simulink model "blocco"  (R2020b)
settings: Solver=VariableStepAuto  StartTime=0.0  StopTime=10.0  RelTol=1e-3
values from neighbouring files (symbols this model uses):
  Beq_hat = 1.07084792335e-06    [params_estimated_LAB0.mat]
  daq =     [params_inertial_case.mat]    (also in params_resonant_case.mat)
  drv =     [params_inertial_case.mat]    (also in params_resonant_case.mat)
  gbox =     [params_inertial_case.mat]    (also in params_resonant_case.mat)
  Jeq_hat = 8.03522579674e-07    [params_estimated_LAB0.mat]
  mot =     [params_inertial_case.mat]    (also in params_resonant_case.mat)
  rads2rpm = 9.54929658551    [params_inertial_case.mat]    (also in params_resonant_case.mat)
  sens =     [params_inertial_case.mat]    (also in params_resonant_case.mat)
  tau_hat = 0.00714370660323    [params_estimated_LAB0.mat]
undefined symbols (not defined in the file or in its folder): ctrl, deg2V, den, pulse2deg, s, V2deg
settings Model: Creator=39345  LastModifiedBy=39345

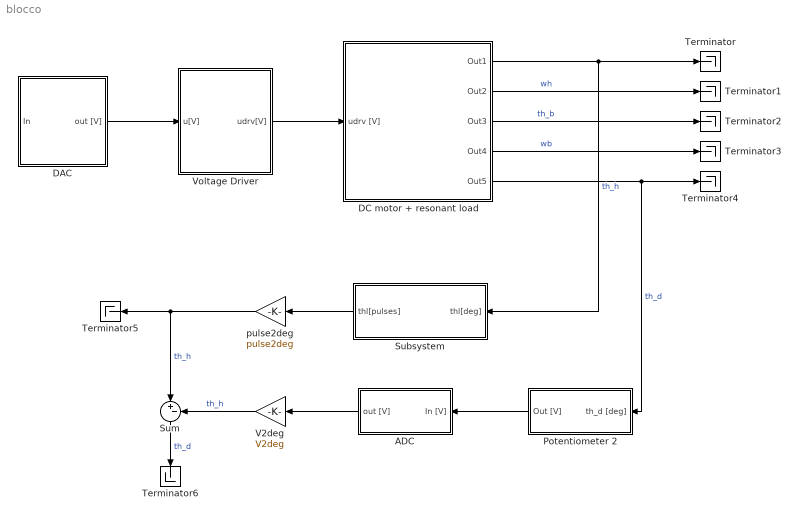
== system blocco ==
  ADC : Subsystem
  DAC : Subsystem
  DC motor + resonant load : Subsystem
  Potentiometer 2 : Subsystem
  Subsystem : Subsystem
  Sum : Sum  Inputs=|+-
  Terminator{,1..6} (7 alike) : Terminator
  V2deg : Gain  Gain=V2deg
  Voltage Driver : Subsystem
  pulse2deg : Gain  Gain=pulse2deg
  wires:
  DC motor + resonant load/1(Out1) -> Subsystem/1(thl[deg]), Terminator/1  "th_h"
  DC motor + resonant load/2(Out2) -> Terminator1/1  "wh"
  DC motor + resonant load/3(Out3) -> Terminator2/1  "th_b"
  DC motor + resonant load/4(Out4) -> Terminator3/1  "wb"
  DC motor + resonant load/5(Out5) -> Potentiometer 2/1(th_d [deg]), Terminator4/1  "th_d"
  Subsystem/1(thl[pulses]) -> pulse2deg/1
  ADC/1(out [V]) -> V2deg/1
  pulse2deg/1 -> Terminator5/1, Sum/1  "th_h"
  V2deg/1 -> Sum/2  "th_h"
  Sum/1 -> Terminator6/1  "th_d"
  DAC/1(out [V]) -> Voltage Driver/1(u[V])
  Voltage Driver/1(udrv[V]) -> DC motor + resonant load/1(udrv [V])
  Potentiometer 2/1(Out [V]) -> ADC/1(In [V])

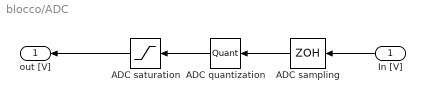
== system blocco/ADC ==
  In [V] : Inport
  ADC quantization : Quantizer  QuantizationInterval=daq.dac.q
  ADC saturation : Saturate  UpperLimit=daq.dac.fs  LowerLimit=-daq.dac.fs
  ADC sampling : ZeroOrderHold  SampleTime=0.001
  out [V] : Outport
  wires:
  ADC saturation/1 -> out [V]/1
  In [V]/1 -> ADC sampling/1
  ADC quantization/1 -> ADC saturation/1
  ADC sampling/1 -> ADC quantization/1

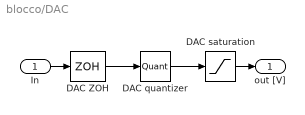
== system blocco/DAC ==
  In : Inport
  DAC quantizer : Quantizer  QuantizationInterval=daq.dac.q
  DAC saturation : Saturate  UpperLimit=daq.dac.fs  LowerLimit=-daq.dac.fs
  DAC ZOH : ZeroOrderHold  SampleTime=0.001
  out [V] : Outport
  wires:
  DAC ZOH/1 -> DAC quantizer/1
  DAC quantizer/1 -> DAC saturation/1
  In/1 -> DAC ZOH/1
  DAC saturation/1 -> out [V]/1

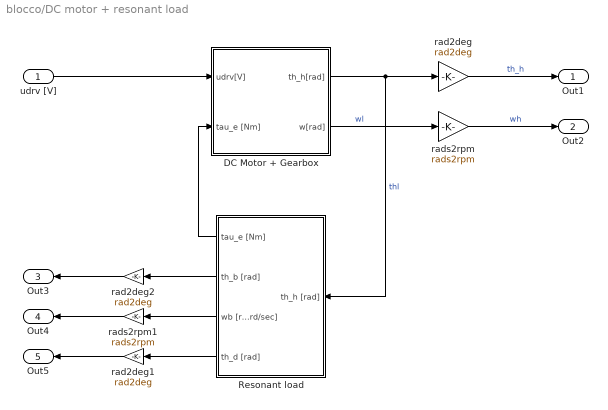
== system blocco/DC motor + resonant load ==
  udrv [V] : Inport
  DC Motor + Gearbox : Subsystem
  Resonant load : Subsystem
  rad2deg : Gain  Gain=rad2deg
  rad2deg1 : Gain  Gain=rad2deg
  rad2deg2 : Gain  Gain=rad2deg
  "rads2rpm " : Gain  Gain=rads2rpm
  "rads2rpm1 " : Gain  Gain=rads2rpm
  Out1 : Outport
  Out2 : Outport  Port=2
  Out3 : Outport  Port=3
  Out4 : Outport  Port=4
  Out5 : Outport  Port=5
  wires:
  Resonant load/3(wb [rard/sec]) -> "rads2rpm1 "/1
  Resonant load/4(th_d [rad]) -> rad2deg1/1
  "rads2rpm1 "/1 -> Out4/1
  rad2deg/1 -> Out1/1  "th_h"
  "rads2rpm "/1 -> Out2/1  "wh"
  rad2deg2/1 -> Out3/1
  udrv [V]/1 -> DC Motor + Gearbox/1(udrv[V])
  Resonant load/2(th_b [rad]) -> rad2deg2/1
  rad2deg1/1 -> Out5/1
  DC Motor + Gearbox/1(th_h[rad]) -> Resonant load/1(th_h [rad]), rad2deg/1  "thl"
  DC Motor + Gearbox/2(w[rad]) -> "rads2rpm "/1  "wl"
  Resonant load/1(tau_e [Nm]) -> DC Motor + Gearbox/2(tau_e [Nm])

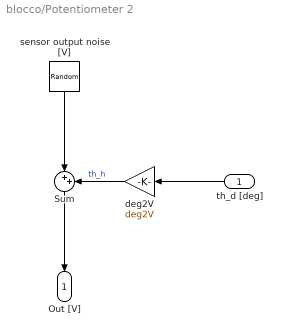
== system blocco/Potentiometer 2 ==
  th_d [deg] : Inport
  Sum : Sum  Inputs=|++
  deg2V : Gain  Gain=deg2V
  "sensor output noise [V] " : RandomNumber  Variance=3.5e-7  SampleTime=0.1
  Out [V] : Outport
  wires:
  th_d [deg]/1 -> deg2V/1
  deg2V/1 -> Sum/2  "th_h"
  "sensor output noise [V] "/1 -> Sum/1
  Sum/1 -> Out [V]/1

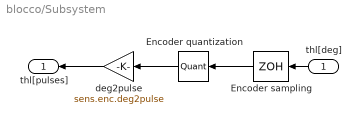
== system blocco/Subsystem ==
  thl[deg] : Inport
  Encoder quantization : Quantizer  QuantizationInterval=sens.enc.pulse2deg
  Encoder sampling : ZeroOrderHold  SampleTime=-1
  deg2pulse : Gain  Gain=sens.enc.deg2pulse
  thl[pulses] : Outport
  wires:
  thl[deg]/1 -> Encoder sampling/1
  Encoder quantization/1 -> deg2pulse/1
  Encoder sampling/1 -> Encoder quantization/1
  deg2pulse/1 -> thl[pulses]/1

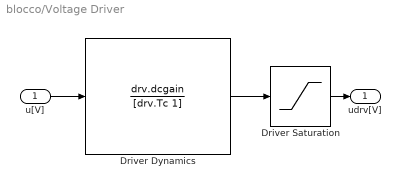
== system blocco/Voltage Driver ==
  u[V] : Inport
  Driver Dynamics : TransferFcn  Numerator=drv.dcgain  Denominator=[drv.Tc 1]
  Driver Saturation : Saturate  UpperLimit=12  LowerLimit=-12
  udrv[V] : Outport
  wires:
  Driver Dynamics/1 -> Driver Saturation/1
  Driver Saturation/1 -> udrv[V]/1
  u[V]/1 -> Driver Dynamics/1

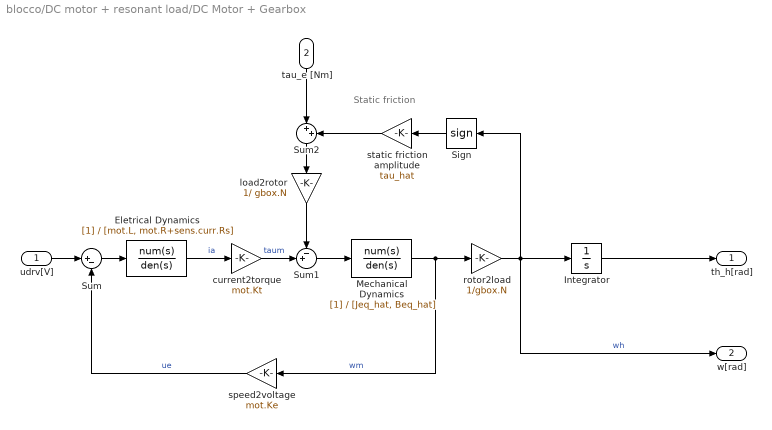
== system blocco/DC motor + resonant load/DC Motor + Gearbox ==
  note: Static friction
  udrv[V] : Inport
  tau_e [Nm] : Inport  Port=2
  Eletrical Dynamics : TransferFcn  Denominator=[mot.L, mot.R+sens.curr.Rs]
  Integrator : Integrator
  Mechanical Dynamics : TransferFcn  Denominator=[Jeq_hat, Beq_hat]
  Sign : Signum  ZeroCross=off
  Sum : Sum  Inputs=|+-
  Sum1 : Sum  Inputs=-+|
  Sum2 : Sum  Inputs=|++
  current2torque : Gain  Gain=mot.Kt
  load2rotor : Gain  Gain=1/ gbox.N
  rotor2load : Gain  Gain=1/gbox.N
  speed2voltage : Gain  Gain=mot.Ke
  static friction amplitude : Gain  Gain=tau_hat
  th_h[rad] : Outport  VectorParamsAs1DForOutWhenUnconnected=off
  w[rad] : Outport  Port=2  VectorParamsAs1DForOutWhenUnconnected=off
  wires:
  Eletrical Dynamics/1 -> current2torque/1  "ia"
  udrv[V]/1 -> Sum/1
  Sum/1 -> Eletrical Dynamics/1
  current2torque/1 -> Sum1/2  "taum"
  Sum1/1 -> Mechanical Dynamics/1
  Mechanical Dynamics/1 -> rotor2load/1, speed2voltage/1  "wm"
  rotor2load/1 -> w[rad]/1, Integrator/1, Sign/1  "wh"
  Integrator/1 -> th_h[rad]/1
  Sign/1 -> static friction amplitude/1
  speed2voltage/1 -> Sum/2  "ue"
  load2rotor/1 -> Sum1/1
  Sum2/1 -> load2rotor/1
  static friction amplitude/1 -> Sum2/2
  tau_e [Nm]/1 -> Sum2/1

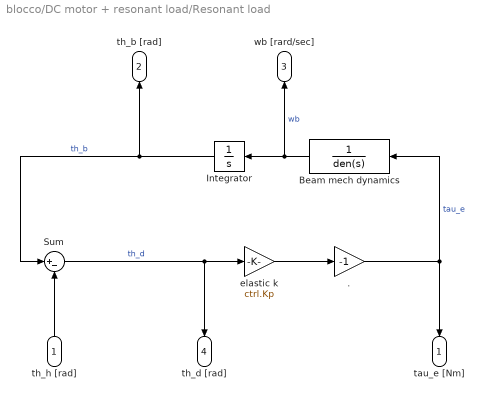
== system blocco/DC motor + resonant load/Resonant load ==
  th_h [rad] : Inport
  . : Gain  Gain=-1
  Beam mech dynamics : TransferFcn  Numerator=[0 1]  Denominator=den(s)
  Integrator : Integrator
  Sum : Sum  Inputs=|+-
  elastic k : Gain  Gain=ctrl.Kp
  tau_e [Nm] : Outport
  th_b [rad] : Outport  Port=2
  wb [rard/sec] : Outport  Port=3
  th_d [rad] : Outport  Port=4
  wires:
  th_h [rad]/1 -> Sum/2
  Sum/1 -> th_d [rad]/1, elastic k/1  "th_d"
  elastic k/1 -> ./1
  ./1 -> Beam mech dynamics/1, tau_e [Nm]/1  "tau_e"
  Beam mech dynamics/1 -> Integrator/1, wb [rard/sec]/1  "wb"
  Integrator/1 -> th_b [rad]/1, Sum/1  "th_b"
